simulink model "Copy_of_FCEvReferenceApplication"  (R2023a)
settings: Solver=ode23t  StartTime=0  StopTime=1369  RelTol=1e-3  EnableMultiTasking=on
libraries: autolibshared x1
settings Model: DataDictionary=VehicleConfig.sldd  ModifiedByFormat=The MathWorks, Inc.  SimulationMode=accelerator  PauseTimes=0  Creator=The MathWorks, Inc.  LastModifiedBy=The MathWorks, Inc.
settings SolverCC: MaxConsecutiveMinStep=12  ZeroCrossAlgorithm=Adaptive  AlgebraicLoopSolver=TrustRegion  AutoInsertRateTranBlk=on  DecoupledContinuousIntegration=on  MinimalZcImpactIntegration=on  MaxZcPerStep=1
settings DataIOCC: SaveOutput=off  DSMLogging=off  SaveTime=off  ReturnWorkspaceOutputs=off
settings OptimizationCC: ReuseModelBlockBuffer=off
settings DebuggingCC: UnderspecifiedInitializationDetection=Classic  MergeDetectMultiDrivingBlocksExec=none  IgnoredZcDiagnostic=none  UnconnectedInputMsg=warning  UnconnectedOutputMsg=warning  UnconnectedLineMsg=warning  ModelReferenceExtraNoncontSigs=none  PregeneratedLibrarySubsystemCodeDiagnostic=none  ArithmeticOperatorsInVariantConditions=warning
settings ModelReferenceCC: UpdateModelReferenceTargets=IfOutOfDate  EnableRefExpFcnMdlSchedulingChecks=on  ModelReferenceMinAlgLoopOccurrences=on  PropagateSignalLabelsOutOfModel=off
settings SFSimCC: SimUseLocalCustomCode=off
settings RTWCC: RTWUseLocalCustomCode=off  Toolchain=Microsoft Visual C++ 2022 v17.0 | CMake/nmake (64-bit Windows)  BuildConfiguration=Release  DLArmComputeVersion=19.05
settings CodeAppCC: StateflowObjectComments=on
settings GRTTargetCC: TargetLangStandard=C89/C90 (ANSI)
settings ConfigComp: CovMetricSettings=dsw  CovSaveCumulativeToWorkspaceVar=on  CovSaveSingleToWorkspaceVar=on  CovExternalEMLEnable=off

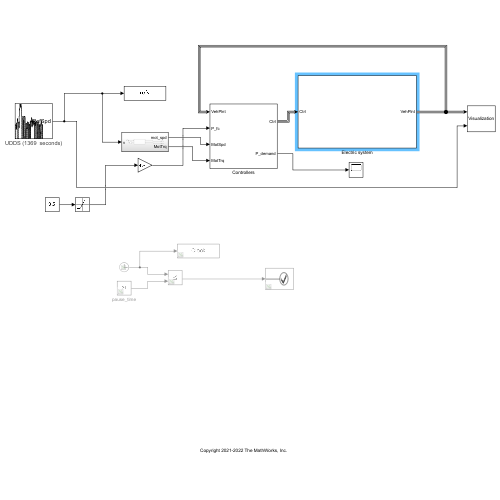
[thumbnail: Simulink's stored preview of the top-level diagram]
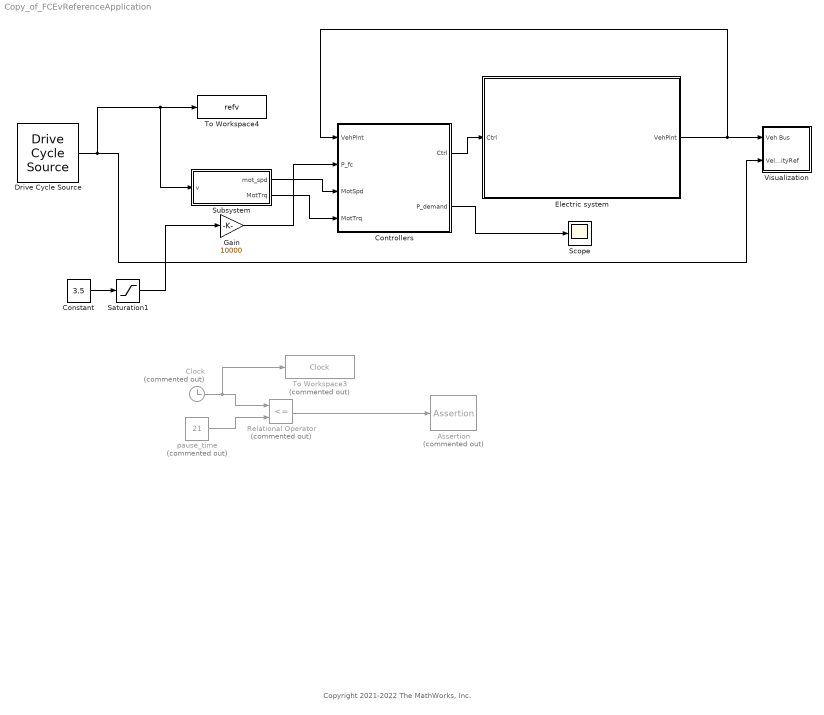
== system Copy_of_FCEvReferenceApplication ==
  note: Copyright 2021-2022 The MathWorks, Inc.
  Assertion : Assertion  Commented=on  AssertionFailFcn=set_param(bdroot, 'SimulationCommand', 'pause')  StopWhenAssertionFail=off
  Clock : Clock  Commented=on
  Constant : Constant  Value=3.5
  Controllers : Subsystem
  Drive Cycle Source : autolibshared/Drive Cycle Source  cycleVar=UDDS  fileVar=L:\Bauto\matlab\test\toolbox\shared\autoblks\scenario\adac.txt  tfinal="1369  seconds"  cycleRepeat=off  outAccPort=off  outGearPort=off  gearList=No gear data  t_wot1=1  xdot_woto=0  xdot_wot1=26.8  t_wot2=30  xdot_wot2=0  t_wotend=40  srcUnit=m/s  outUnit=m/s  srcAccUnit=m/s/s  outAccUnit=m/s^2  dt=0  aMode=1  faultOption=off  velBnd=2  velBndUnit=mph  inUnit=m/s  timeBnd=1  failOption=off  stopSim=off  maxFaultCnt=10  maxFaultTime=2  maxTotFaultTime=15  traceOption=off  dtTrace=1  traceWindow=10  lastDCname=UDDS  lastOutUnit=mph  lastDT=0  lastTB=1  lastSB=2  forceCalcBound=off
  Electric system : Subsystem
  Gain : Gain  Gain=10000
  Relational Operator : RelationalOperator  Commented=on  Operator=<=  OutDataTypeStr=boolean  RndMeth=Simplest  InputSameDT=off
  Saturation1 : Saturate  UpperLimit=35  LowerLimit=0
  Scope : Scope
  Subsystem : Subsystem
  To Workspace3 : ToWorkspace  Commented=on  VariableName=Clock  SampleTime=1
  To Workspace4 : ToWorkspace  VariableName=refv  SampleTime=1
  Visualization : Subsystem
      mask Display: disp(getString(message('autoblks:autoblkVehMask:visual')))
  pause_time : Constant  Commented=on  Value=21
  wires:
  Controllers/1(Ctrl) -> Electric system/1(Ctrl)
  Electric system/1(VehPlnt) -> Controllers/1(VehPlnt), Visualization/1(Veh Bus)
  Controllers/2(P_demand) -> Scope/1
  pause_time/1 -> Relational Operator/2
  Clock/1 -> To Workspace3/1, Relational Operator/1
  Relational Operator/1 -> Assertion/1
  Gain/1 -> Controllers/2(P_fc)
  Constant/1 -> Saturation1/1
  Saturation1/1 -> Gain/1
  Subsystem/1(mot_spd) -> Controllers/3(MotSpd)
  Subsystem/2(MotTrq) -> Controllers/4(MotTrq)
  Drive Cycle Source/1 -> Subsystem/1(v), To Workspace4/1, Visualization/2(VelocityRef)

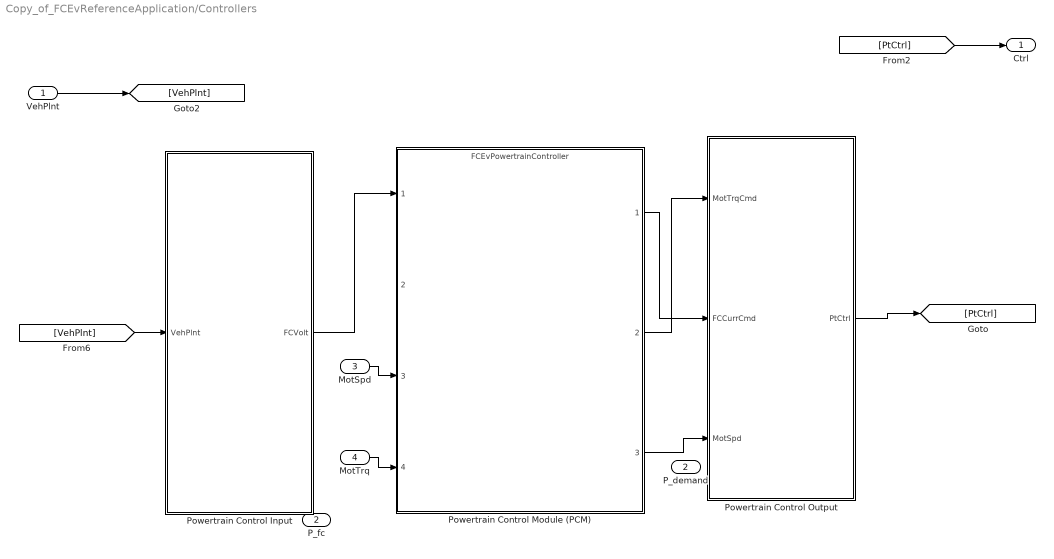
== system Copy_of_FCEvReferenceApplication/Controllers ==
  VehPlnt : Inport
  P_fc : Inport  Port=2
  MotSpd : Inport  Port=3
  MotTrq : Inport  Port=4
  Powertrain Control Input : Subsystem
  Powertrain Control Module (PCM) : ModelReference  ModelNameDialog=FCEvPowertrainController.slx  ModelReferenceVersion=6.21
  Powertrain Control Output : Subsystem
  Ctrl : Outport  VectorParamsAs1DForOutWhenUnconnected=off
  P_demand : Outport  Port=2
  wires:
  VehPlnt/1 -> [VehPlnt]
  [PtCtrl] -> Ctrl/1
  [VehPlnt] -> Powertrain Control Input/1(VehPlnt)
  Powertrain Control Output/1(PtCtrl) -> [PtCtrl]
  Powertrain Control Input/1(FCVolt) -> Powertrain Control Module (PCM)/1
  Powertrain Control Module (PCM)/1 -> Powertrain Control Output/2(FCCurrCmd)
  Powertrain Control Module (PCM)/3 -> Powertrain Control Output/3(MotSpd)
  MotTrq/1 -> Powertrain Control Module (PCM)/4
  MotSpd/1 -> Powertrain Control Module (PCM)/3
  Powertrain Control Module (PCM)/2 -> Powertrain Control Output/1(MotTrqCmd)
  ? -> P_demand/1

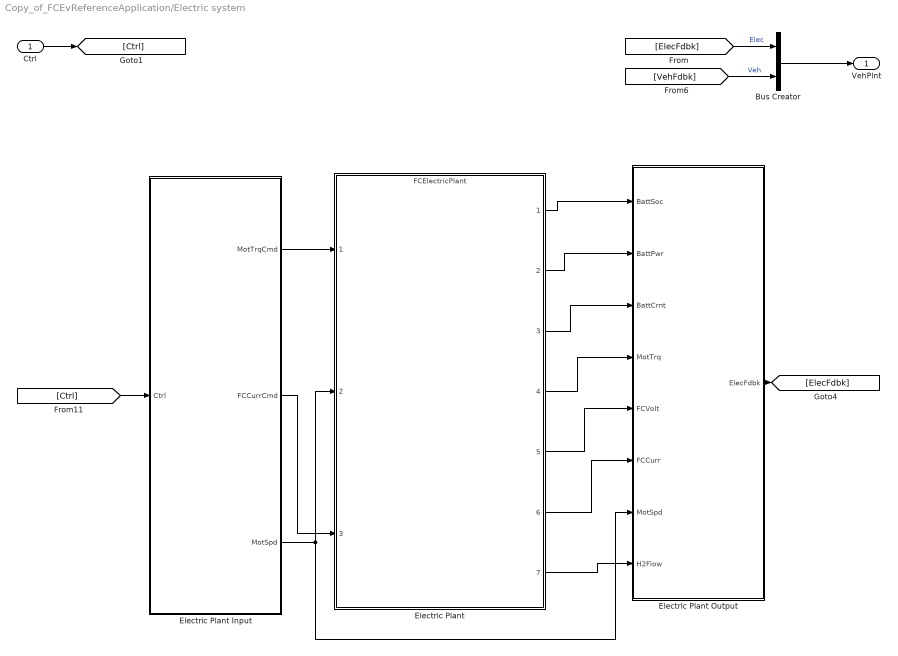
== system Copy_of_FCEvReferenceApplication/Electric system ==
  Ctrl : Inport
  Bus Creator : BusCreator  Inputs=2
  Electric Plant : ModelReference  ModelNameDialog=FCElectricPlant.slx  ModelReferenceVersion=6.19
  Electric Plant Input : Subsystem
  Electric Plant Output : Subsystem
  VehPlnt : Outport  VectorParamsAs1DForOutWhenUnconnected=off
  wires:
  Electric Plant/1 -> Electric Plant Output/1(BattSoc)
  Electric Plant/6 -> Electric Plant Output/6(FCCurr)
  Electric Plant/5 -> Electric Plant Output/5(FCVolt)
  Electric Plant/3 -> Electric Plant Output/3(BattCrnt)
  Electric Plant/4 -> Electric Plant Output/4(MotTrq)
  Bus Creator/1 -> VehPlnt/1
  [ElecFdbk] -> Bus Creator/1  "Elec"
  Electric Plant Output/1(ElecFdbk) -> [ElecFdbk]
  Electric Plant Input/1(MotTrqCmd) -> Electric Plant/1
  Electric Plant/2 -> Electric Plant Output/2(BattPwr)
  [VehFdbk] -> Bus Creator/2  "Veh"
  [Ctrl] -> Electric Plant Input/1(Ctrl)
  Ctrl/1 -> [Ctrl]
  Electric Plant Input/2(FCCurrCmd) -> Electric Plant/3
  Electric Plant Input/3(MotSpd) -> Electric Plant Output/7(MotSpd), Electric Plant/2
  Electric Plant/7 -> Electric Plant Output/8(H2Flow)

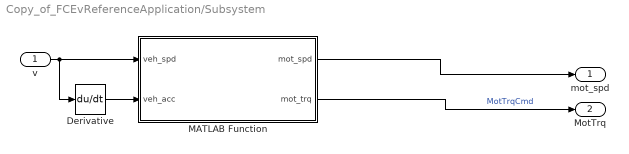
== system Copy_of_FCEvReferenceApplication/Subsystem ==
  v : Inport
  Derivative : Derivative
  MATLAB Function : MATLAB Function  TreatAsAtomicUnit=on
  mot_spd : Outport
  MotTrq : Outport  Port=2
  wires:
  v/1 -> Derivative/1, MATLAB Function/1(veh_spd)
  MATLAB Function/1(mot_spd) -> mot_spd/1
  MATLAB Function/2(mot_trq) -> MotTrq/1  "MotTrqCmd"
  Derivative/1 -> MATLAB Function/2(veh_acc)

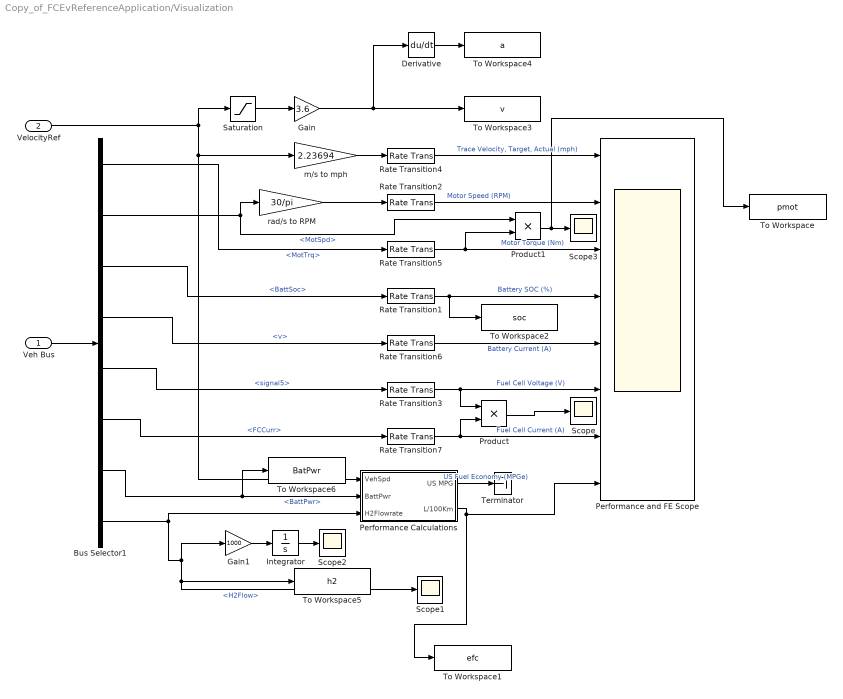
== system Copy_of_FCEvReferenceApplication/Visualization ==
  Veh Bus : Inport
  VelocityRef : Inport  Port=2
  Bus Selector1 : BusSelector  OutputSignals=Elec.MotTrq,Elec.MotSpd,Elec.BattSoc,Elec.v,Elec.signal5,Elec.FCCurr,Elec.BattPwr,Elec.H2Flow
  Derivative : Derivative
  Gain : Gain  Gain=3.6
  Gain1 : Gain  Gain=1000
  Integrator : Integrator
  Performance Calculations : Subsystem
  Performance and FE Scope : Scope  NumInputPorts=8
  Product : Product
  Product1 : Product
  Rate Transition{1..7} (7 alike) : RateTransition  Deterministic=off
  Saturation : Saturate  UpperLimit=Inf  LowerLimit=0
  Scope{,1..3} (4 alike) : Scope
  Terminator : Terminator
  To Workspace : ToWorkspace  VariableName=pmot  SampleTime=1
  To Workspace1 : ToWorkspace  VariableName=efc  SampleTime=1
  To Workspace2 : ToWorkspace  VariableName=soc  SampleTime=1
      settings: Save2DSignal=2-D array (concatenate along first dimension)
  To Workspace3 : ToWorkspace  VariableName=v  SampleTime=1
  To Workspace4 : ToWorkspace  VariableName=a  SampleTime=1
  To Workspace5 : ToWorkspace  VariableName=h2  SampleTime=1
  To Workspace6 : ToWorkspace  VariableName=BatPwr  SampleTime=1
      settings: Save2DSignal=2-D array (concatenate along first dimension)
  m/s to mph : Gain  Gain=2.23694
  rad/s to RPM : Gain  Gain=30/pi
  wires:
  Veh Bus/1 -> Bus Selector1/1
  VelocityRef/1 -> Performance Calculations/1(VehSpd), m/s to mph/1, Saturation/1
  Performance Calculations/2(L/100Km) -> Performance and FE Scope/8, To Workspace1/1
  m/s to mph/1 -> Rate Transition4/1
  Bus Selector1/3 -> Rate Transition1/1  "<BattSoc>"
  Rate Transition1/1 -> To Workspace2/1, Performance and FE Scope/4  "Battery SOC (%)"
  Rate Transition2/1 -> Performance and FE Scope/2  "Motor Speed (RPM)"
  Rate Transition4/1 -> Performance and FE Scope/1  "Trace Velocity, Target, Actual (mph)"
  Bus Selector1/2 -> rad/s to RPM/1, Product1/1  "<MotSpd>"
  Bus Selector1/7 -> To Workspace6/1, Performance Calculations/2(BattPwr)  "<BattPwr>"
  rad/s to RPM/1 -> Rate Transition2/1
  Bus Selector1/1 -> Rate Transition5/1  "<MotTrq>"
  Rate Transition5/1 -> Product1/2, Performance and FE Scope/3  "Motor Torque (Nm)"
  Rate Transition6/1 -> Performance and FE Scope/5  "Battery Current (A)"
  Bus Selector1/4 -> Rate Transition6/1  "<v>"
  Bus Selector1/8 -> Performance Calculations/3(H2Flowrate), To Workspace5/1, Scope1/1, Gain1/1  "<H2Flow>"
  Bus Selector1/6 -> Rate Transition7/1  "<FCCurr>"
  Rate Transition7/1 -> Performance and FE Scope/7, Product/2  "Fuel Cell Current (A)"
  Bus Selector1/5 -> Rate Transition3/1  "<signal5>"
  Rate Transition3/1 -> Performance and FE Scope/6, Product/1  "Fuel Cell Voltage (V)"
  Product/1 -> Scope/1
  Saturation/1 -> Gain/1
  Gain/1 -> Derivative/1, To Workspace3/1
  Derivative/1 -> To Workspace4/1
  Integrator/1 -> Scope2/1
  Gain1/1 -> Integrator/1
  Performance Calculations/1(US MPG) -> Terminator/1  "US Fuel Economy (MPGe)"
  Product1/1 -> To Workspace/1, Scope3/1

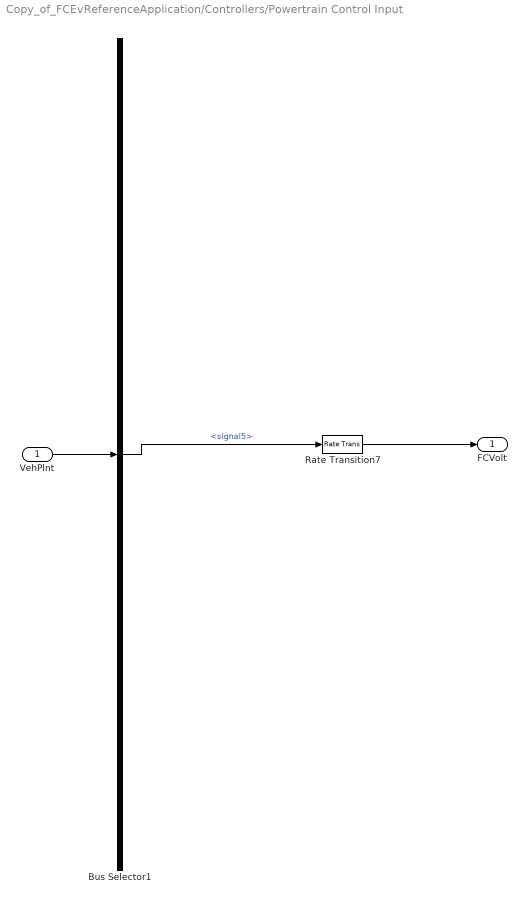
== system Copy_of_FCEvReferenceApplication/Controllers/Powertrain Control Input ==
  VehPlnt : Inport
  Bus Selector1 : BusSelector  OutputSignals=Elec.signal5
  Rate Transition7 : RateTransition  Deterministic=off
  FCVolt : Outport  VectorParamsAs1DForOutWhenUnconnected=off
  wires:
  VehPlnt/1 -> Bus Selector1/1
  Rate Transition7/1 -> FCVolt/1
  Bus Selector1/1 -> Rate Transition7/1  "<signal5>"

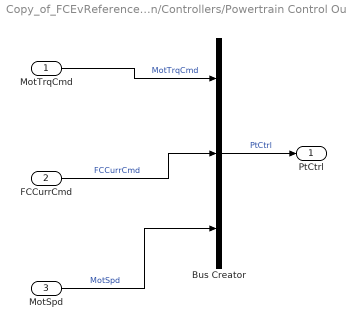
== system Copy_of_FCEvReferenceApplication/Controllers/Powertrain Control Output ==
  MotTrqCmd : Inport
  FCCurrCmd : Inport  Port=2
  MotSpd : Inport  Port=3
  Bus Creator : BusCreator  Inputs=3
  PtCtrl : Outport  VectorParamsAs1DForOutWhenUnconnected=off
  wires:
  Bus Creator/1 -> PtCtrl/1  "PtCtrl"
  MotTrqCmd/1 -> Bus Creator/1  "MotTrqCmd"
  FCCurrCmd/1 -> Bus Creator/2  "FCCurrCmd"
  MotSpd/1 -> Bus Creator/3  "MotSpd"

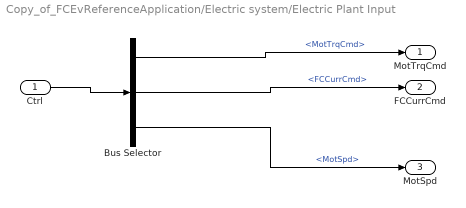
== system Copy_of_FCEvReferenceApplication/Electric system/Electric Plant Input ==
  Ctrl : Inport
  Bus Selector : BusSelector  OutputSignals=MotTrqCmd,FCCurrCmd,MotSpd
  MotTrqCmd : Outport  VectorParamsAs1DForOutWhenUnconnected=off
  FCCurrCmd : Outport  Port=2  VectorParamsAs1DForOutWhenUnconnected=off
  MotSpd : Outport  Port=3  VectorParamsAs1DForOutWhenUnconnected=off
  wires:
  Ctrl/1 -> Bus Selector/1
  Bus Selector/1 -> MotTrqCmd/1  "<MotTrqCmd>"
  Bus Selector/2 -> FCCurrCmd/1  "<FCCurrCmd>"
  Bus Selector/3 -> MotSpd/1  "<MotSpd>"

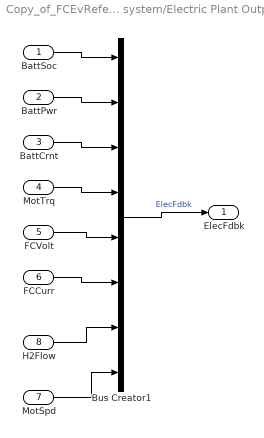
== system Copy_of_FCEvReferenceApplication/Electric system/Electric Plant Output ==
  BattSoc : Inport
  BattPwr : Inport  Port=2
  BattCrnt : Inport  Port=3
  MotTrq : Inport  Port=4
  FCVolt : Inport  Port=5
  FCCurr : Inport  Port=6
  MotSpd : Inport  Port=7
  H2Flow : Inport  Port=8
  Bus Creator1 : BusCreator  Inputs=8
  ElecFdbk : Outport  VectorParamsAs1DForOutWhenUnconnected=off
  wires:
  Bus Creator1/1 -> ElecFdbk/1  "ElecFdbk"
  BattPwr/1 -> Bus Creator1/2
  BattSoc/1 -> Bus Creator1/1
  BattCrnt/1 -> Bus Creator1/3
  MotTrq/1 -> Bus Creator1/4
  FCVolt/1 -> Bus Creator1/5
  FCCurr/1 -> Bus Creator1/6
  H2Flow/1 -> Bus Creator1/7
  MotSpd/1 -> Bus Creator1/8

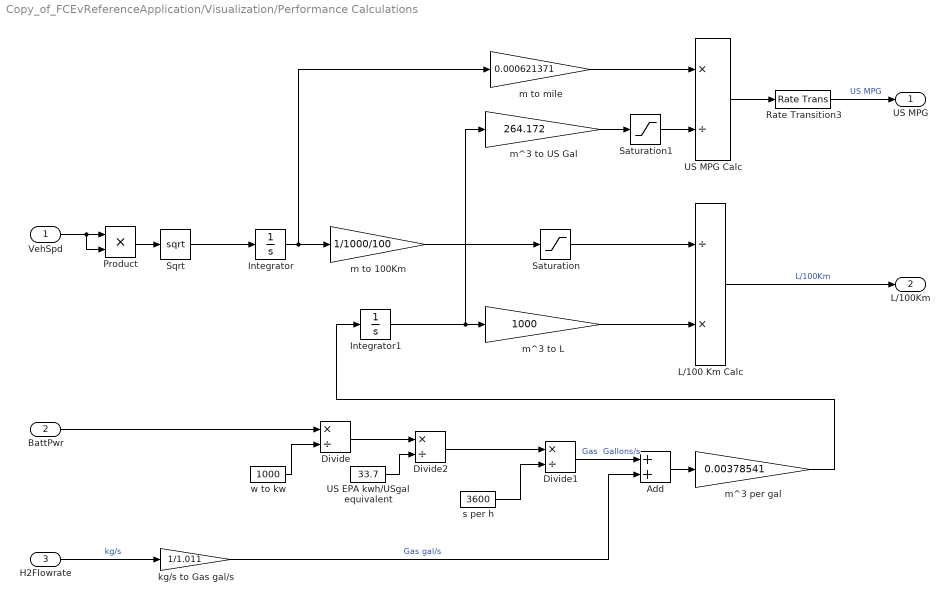
== system Copy_of_FCEvReferenceApplication/Visualization/Performance Calculations ==
  VehSpd : Inport
  BattPwr : Inport  Port=2
  H2Flowrate : Inport  Port=3
  Add : Sum
  Divide : Product  Inputs=*/
  Divide1 : Product  Inputs=*/
  Divide2 : Product  Inputs=*/
  Integrator : Integrator
  Integrator1 : Integrator
  L/100 Km Calc : Product  Inputs=/*
  Product : Product
  Rate Transition3 : RateTransition  Deterministic=off
  Saturation : Saturate  UpperLimit=Inf  LowerLimit=0.001
  Saturation1 : Saturate  UpperLimit=Inf  LowerLimit=1e-3
  Sqrt : Sqrt
  US EPA kwh/USgal equivalent : Constant  Value=33.7
  US MPG Calc : Product  Inputs=*/
  kg/s to Gas gal/s : Gain  Gain=1/1.011
  m to 100Km : Gain  Gain=1/1000/100
  m to mile : Gain  Gain=0.000621371
  m^3 per gal : Gain  Gain=0.00378541
  m^3 to L : Gain  Gain=1000
  m^3 to US Gal : Gain  Gain=264.172
  s per h : Constant  Value=3600
  w to kw : Constant  Value=1000
  US MPG : Outport  VectorParamsAs1DForOutWhenUnconnected=off
  L/100Km : Outport  Port=2  VectorParamsAs1DForOutWhenUnconnected=off
  wires:
  m^3 to US Gal/1 -> Saturation1/1
  m^3 to L/1 -> L/100 Km Calc/2
  Integrator/1 -> m to mile/1, m to 100Km/1
  m to mile/1 -> US MPG Calc/1
  Integrator1/1 -> m^3 to US Gal/1, m^3 to L/1
  Saturation/1 -> L/100 Km Calc/1
  m to 100Km/1 -> Saturation/1
  L/100 Km Calc/1 -> L/100Km/1  "L/100Km"
  US MPG Calc/1 -> Rate Transition3/1
  Saturation1/1 -> US MPG Calc/2
  Rate Transition3/1 -> US MPG/1  "US MPG"
  w to kw/1 -> Divide/2
  Divide/1 -> Divide2/1
  Divide2/1 -> Divide1/1
  s per h/1 -> Divide1/2
  Divide1/1 -> Add/1  "Gas  Gallons/s"
  US EPA kwh/USgal equivalent/1 -> Divide2/2
  BattPwr/1 -> Divide/1
  Sqrt/1 -> Integrator/1
  Product/1 -> Sqrt/1
  VehSpd/1 -> Product/2, Product/1
  m^3 per gal/1 -> Integrator1/1
  H2Flowrate/1 -> kg/s to Gas gal/s/1  "kg/s"
  kg/s to Gas gal/s/1 -> Add/2  "Gas gal/s"
  Add/1 -> m^3 per gal/1

== matlab function Copy_of_FCEvReferenceApplication/Subsystem/MATLAB Function ==
  data: mot_spd output; veh_spd input; mot_trq output; veh_acc input
function [mot_spd,mot_trq] = fcn(veh_spd,veh_acc)
veh_whl_radius = 0.327;
veh_mass = 1500;
veh_rrc  = 0.015;
veh_air_density = 1.2;
veh_FA = 2.27;
veh_CD = 0.28;
veh_gravity = 9.81;
veh_fd_ratio = 7.94;

w_whl = veh_spd ./ veh_whl_radius;
F_roll = (veh_spd > 0) .* veh_mass .* veh_gravity .* veh_rrc;
F_drag = 0.5 .* veh_air_density .* veh_FA .* veh_CD .* (veh_spd.^2);
F_acc = veh_mass .* veh_acc;
T_whl = veh_whl_radius .* (F_acc + F_roll + F_drag);
mot_t = T_whl./veh_fd_ratio;
mot_trq = mot_t;
mot_spd = w_whl.*veh_fd_ratio;
